simulink model "Mpc_SimMechanics_with_standing"  (R2017b)
settings: Solver=ode45  StartTime=0  StopTime=10  FixedStep=0.0005  EnableMultiTasking=on
InitFcn:
  | isSim = 1;
  | 
  | PreFunctions.CustomInitFcn_with_standing;
  | PreFunctions.simulationInitFcn_with_standing;
undefined symbols (not defined in the file): alpha_x, alpha_y, DiagnosticCodes, DynamicMatrixLibrary, motorPositions, motorVelocities, pelvisPosition, pelvisVelocity, sample_time, X, Y, Z
libraries: sm_lib x170, nesl_utility x75, Contact_Forces_Lib x6, ComponentLibrary x5, xpcrtudplib x2, slrtlib x1
(part 2 of 8)

== system Mpc_SimMechanics_with_standing/Cassie/Cassie Simulation ==
  Bus Element In2 : Inport  PortName=InBus  Element=leftLeg
  Bus Element In3 : Inport  PortName=InBus  Element=rightLeg
  Bus Element In1 : Inport  PortName=InBus  Element=pelvis
  Cassie Left Leg : Subsystem  AncestorBlock=CassieLibrary/Simulation/Cassie Leg  mask{config=Left, motorPositions=motorPositions(1:5), motorVelocities=motorVelocities(1:5)}
      mask prompts: config "Configuration:"; motorPositions "Initial Motor Positions (rad):"; motorVelocities "Initial Motor Velocities (rad/s):"
      mask init:
      | d = CassieDescriptor;
      | bodyIndex = @(s, name) find(arrayfun(@(s) isequal(s.name, name), s));
      | 
      | switch config
      |   case 1 % Left
      |     % Hip Roll
      |     b = d(bodyIndex(d, 'left-hip-roll'));
      |     set_param([gcb, '/Hip Roll Solid'], 'ExtGeomFileName', [b.name '.stl']);
      |     set_param([gcb, '/Hip Roll Solid'], 'Mass', mat2str(b.m));
      |     set_param([gcb, '/Hip Roll Solid'], 'CenterOfMass', mat2str(b.c));
      |     set_param([gcb, '/Hip Roll Solid'], 'MomentsOfInertia', mat2str(b.Ic(1:3)));
      |     set_param([gcb, '/Hip Roll Solid'], 'ProductsOfInertia', mat2str(b.Ic(4:6)));
      |     %set_param([gcb, '/Pelvis to Hip Roll'], 'TranslationCartesianOffset', mat2str(b.r));
      |     %set_param([gcb, '/Pelvis to Hip Roll'], 'RotationMatrix', mat2str(b.R));
      |     
      |     % Hip Yaw
      |     b = d(bodyIndex(d, 'left-hip-yaw'));
      |     set_param([gcb, '/Hip Yaw Solid'], 'ExtGeomFileName', [b.name '.stl']);
      |     set_param([gcb, '/Hip Yaw Solid'], 'Mass', mat2str(b.m));
      |     set_param([gcb, '/Hip Yaw Solid'], 'CenterOfMass', mat2str(b.c));
      |     set_param([gcb, '/Hip Yaw Solid'], 'MomentsOfInertia', mat2str(b.Ic(1:3)));
      |     set_param([gcb, '/Hip Yaw Solid'], 'ProductsOfInertia', mat2str(b.Ic(4:6)));
      |     set_param([gcb, '/Hip Roll to Hip Yaw'], 'TranslationCartesianOffset', mat2str(b.r));
      |     set_param([gcb, '/Hip Roll to Hip Yaw'], 'RotationMatrix', mat2str(b.R));
      |     
      |     % Hip Pitch
      |     b = d(bodyIndex(d, 'left-hip-pitch'));
      |     set_param([gcb, '/Hip Pitch Solid'], 'ExtGeomFileName', [b.name '.stl']);
      |     set_param([gcb, '/Hip Pitch Solid'], 'Mass', mat2str(b.m));
      |     set_param([gcb, '/Hip Pitch Solid'], 'CenterOfMass', mat2str(b.c));
      |     set_param([gcb, '/Hip Pitch Solid'], 'MomentsOfInertia', mat2str(b.Ic(1:3)));
      |     set_param([gcb, '/Hip Pitch Solid'], 'ProductsOfInertia', mat2str(b.Ic(4:6)));
      |     set_param([gcb, '/Hip Yaw to Hip Pitch'], 'TranslationCartesianOffset', mat2str(b.r));
      |     set_param([gcb, '/Hip Yaw to Hip Pitch'], 'RotationMatrix', mat2str(b.R));
      |     
      |     % Achilles Rod
      |     b = d(bodyIndex(d, 'left-achilles-rod'));
      |     set_param([gcb, '/Achilles Rod Solid'], 'ExtGeomFileName', [b.name '.stl']);
      |     set_param([gcb, '/Achilles Rod Solid'], 'Mass', mat2str(b.m));
      |     set_param([gcb, '/Achilles Rod Solid'], 'CenterOfMass', mat2str(b.c));
      |     set_param([gcb, '/Achilles Rod Solid'], 'MomentsOfInertia', mat2str(b.Ic(1:3)));
      |     set_param([gcb, '/Achilles Rod Solid'], 'ProductsOfInertia', mat2str(b.Ic(4:6)));
      |     set_param([gcb, '/Hip Pitch to Achilles Rod'], 'TranslationCartesianOffset', mat2str(b.r));
      |     set_param([gcb, '/Hip Pitch to Achilles Rod'], 'RotationMatrix', mat2str(b.R));
      |     
      |     % Knee
      |     b = d(bodyIndex(d, 'left-knee'));
      |     set_param([gcb, '/Knee Solid'], 'ExtGeomFileName', [b.name '.stl']);
      |     set_param([gcb, '/Knee Solid'], 'Mass', mat2str(b.m));
      |     set_param([gcb, '/Knee Solid'], 'CenterOfMass', mat2str(b.c));
      |     set_param([gcb, '/Knee Solid'], 'MomentsOfInertia', mat2str(b.Ic(1:3)));
      |     set_param([gcb, '/Knee Solid'], 'ProductsOfInertia', mat2str(b.Ic(4:6)));
      |     set_param([gcb, '/Hip Pitch to Knee'], 'TranslationCartesianOffset', mat2str(b.r));
      |     set_param([gcb, '/Hip Pitch to Knee'], 'RotationMatrix', mat2str(b.R));
      |     
      |     % Knee Spring
      |     b = d(bodyIndex(d, 'left-knee-spring'));
      |     set_param([gcb, '/Knee Spring Solid'], 'ExtGeomFileName', [b.name '.stl']);
      |     set_param([gcb, '/Knee Spring Solid'], 'Mass', mat2str(b.m));
      |     set_param([gcb, '/Knee Spring Solid'], 'CenterOfMass', mat2str(b.c));
      |     set_param([gcb, '/Knee Spring Solid'], 'MomentsOfInertia', mat2str(b.Ic(1:3)));
      |     set_param([gcb, '/Knee Spring Solid'], 'ProductsOfInertia', mat2str(b.Ic(4:6)));
      |     set_param([gcb, '/Knee to Knee Spring'], 'TranslationCartesianOffset', mat2str(b.r));
      |     set_param([gcb, '/Knee to Knee Spring'], 'RotationMatrix', mat2str(b.R));
      |     
      |     % Shin
      |     b = d(bodyIndex(d, 'left-shin'));
      |     set_param([gcb, '/Shin Solid'], 'ExtGeomFileName', [b.name '.stl']);
      |     set_param([gcb, '/Shin Solid'], 'Mass', mat2str(b.m));
      |     set_param([gcb, '/Shin Solid'], 'CenterOfMass', mat2str(b.c));
      |     set_param([gcb, '/Shin Solid'], 'MomentsOfInertia', mat2str(b.Ic(1:3)));
      |     set_param([gcb, '/Shin Solid'], 'ProductsOfInertia', mat2str(b.Ic(4:6)));
      |     set_param([gcb, '/Knee to Shin'], 'TranslationCartesianOffset', mat2str(b.r));
      |     set_param([gcb, '/Knee to Shin'], 'RotationMatrix', mat2str(b.R));
      |     
      |     % Tarsus
      |     b = d(bodyIndex(d, 'left-tarsus'));
      |     set_param([gcb, '/Tarsus Solid'], 'ExtGeomFileName', [b.name '.stl']);
      |     set_param([gcb, '/Tarsus Solid'], 'Mass', mat2str(b.m));
      |     set_param([gcb, '/Tarsus Solid'], 'CenterOfMass', mat2str(b.c));
      |     set_param([gcb, '/Tarsus Solid'], 'MomentsOfInertia', mat2str(b.Ic(1:3)));
      |     set_param([gcb, '/Tarsus Solid'], 'ProductsOfInertia', mat2str(b.Ic(4:6)));
      |     set_param([gcb, '/Shin to Tarsus'], 'TranslationCartesianOffset', mat2str(b.r));
      |     set_param([gcb, '/Shin to Tarsus'], 'RotationMatrix', mat2str(b.R));
      |     
      |     % Heel Spring
      |     b = d(bodyIndex(d, 'left-heel-spring'));
      |     set_param([gcb, '/Heel Spring Solid'], 'ExtGeomFileName', [b.name '.stl']);
      |     set_param([gcb, '/Heel Spring Solid'], 'Mass', mat2str(b.m));
      |     set_param([gcb, '/Heel Spring Solid'], 'CenterOfMass', mat2str(b.c));
      |     set_param([gcb, '/Heel Spring Solid'], 'MomentsOfInertia', mat2str(b.Ic(1:3)));
      |     set_param([gcb, '/Heel Spring Solid'], 'ProductsOfInertia', mat2str(b.Ic(4:6)));
      |     set_param([gcb, '/Tarsus to Heel Spring'], 'TranslationCartesianOffset', mat2str(b.r));
      |     set_param([gcb, '/Tarsus to Heel Spring'], 'RotationMatrix', mat2str(b.R));
      |     
      |     % Foot Crank
      |     b = d(bodyIndex(d, 'left-foot-crank'));
      |     set_param([gcb, '/Foot Crank Solid'], 'ExtGeomFileName', [b.name '.stl']);
      |     set_param([gcb, '/Foot Crank Solid'], 'Mass', mat2str(b.m));
      |     set_param([gcb, '/Foot Crank Solid'], 'CenterOfMass', mat2str(b.c));
      |     set_param([gcb, '/Foot Crank Solid'], 'MomentsOfInertia', mat2str(b.Ic(1:3)));
      |     set_param([gcb, '/Foot Crank Solid'], 'ProductsOfInertia', mat2str(b.Ic(4:6)));
      |     set_param([gcb, '/Tarsus to Foot Crank'], 'TranslationCartesianOffset', mat2str(b.r));
      |     set_param([gcb, '/Tarsus to Foot Crank'], 'RotationMatrix', mat2str(b.R));
      |     
      |     % Plantar Rod
      |     b = d(bodyIndex(d, 'left-plantar-rod'));
      |     set_param([gcb, '/Plantar Rod Solid'], 'ExtGeomFileName', [b.name '.stl']);
      |     set_param([gcb, '/Plantar Rod Solid'], 'Mass', mat2str(b.m));
      |     set_param([gcb, '/Plantar Rod Solid'], 'CenterOfMass', mat2str(b.c));
      |     set_param([gcb, '/Plantar Rod Solid'], 'MomentsOfInertia', mat2str(b.Ic(1:3)));
      |     set_param([gcb, '/Plantar Rod Solid'], 'ProductsOfInertia', mat2str(b.Ic(4:6)));
      |     set_param([gcb, '/Foot Crank to Plantar Rod'], 'TranslationCartesianOffset', mat2str(b.r));
      |     set_param([gcb, '/Foot Crank to Plantar Rod'], 'RotationMatrix', mat2str(b.R));
      |     
      |     % Foot
      |     b = d(bodyIndex(d, 'left-foot'));
      |     set_param([gcb, '/Foot Solid'], 'ExtGeomFileName', [b.name '.stl']);
      |     set_param([gcb, '/Foot Solid'], 'Mass', mat2str(b.m));
      |     set_param([gcb, '/Foot Solid'], 'CenterOfMass', mat2str(b.c));
      |     set_param([gcb, '/Foot Solid'], 'MomentsOfInertia', mat2str(b.Ic(1:3)));
      |     set_param([gcb, '/Foot Solid'], 'ProductsOfInertia', mat2str(b.Ic(4:6)));
      |     set_param([gcb, '/Tarsus to Foot'], 'TranslationCartesianOffset', mat2str(b.r));
      |     set_param([gcb, '/Tarsus to Foot'], 'RotationMatrix', mat2str(b.R));
      |     
      |     % Foot Pin
      |     %b = d(bodyIndex(d, 'left-foot-pin'));
      |     set_param([gcb, '/Foot to Foot Pin'], 'TranslationCartesianOffset', mat2str([0.055 0 0.00776]));
      |     set_param([gcb, '/Foot to Foot Pin'], 'RotationMatrix', mat2str(eye(3)));
      |     
      |     % Midfoot
      |     %b = d(bodyIndex(d, 'left-mid-foot'));
      |     set_param([gcb, '/Foot to Midfoot'], 'TranslationCartesianOffset', mat2str([0.01762 0.05219 0]));
      |     set_param([gcb, '/Foot to Midfoot'], 'RotationMatrix', mat2str([-0.766044443118978 0 -0.642787609686539;0.642787609686539 0 -0.766044443118978;0 -1 0]));
      |     
      |   case 2 % Right
      |     % Hip Roll
      |     b = d(bodyIndex(d, 'right-hip-roll'));
      |     set_param([gcb, '/Hip Roll Solid'], 'ExtGeomFileName', [b.name '.stl']);
      |     set_param([gcb, '/Hip Roll Solid'], 'Mass', mat2str(b.m));
      |     set_param([gcb, '/Hip Roll Solid'], 'CenterOfMass', mat2str(b.c));
      |     set_param([gcb, '/Hip Roll Solid'], 'MomentsOfInertia', mat2str(b.Ic(1:3)));
      |     set_param([gcb, '/Hip Roll Solid'], 'ProductsOfInertia', mat2str(b.Ic(4:6)));
      |     %set_param([gcb, '/Pelvis to Hip Roll'], 'TranslationCartesianOffset', mat2str(b.r));
      |     %set_param([gcb, '/Pelvis to Hip Roll'], 'RotationMatrix', mat2str(b.R));
      |     
      |     % Hip Yaw
      |     b = d(bodyIndex(d, 'right-hip-yaw'));
      |     set_param([gcb, '/Hip Yaw Solid'], 'ExtGeomFileName', [b.name '.stl']);
      |     set_param([gcb, '/Hip Yaw Solid'], 'Mass', mat2str(b.m));
      |     set_param([gcb, '/Hip Yaw Solid'], 'CenterOfMass', mat2str(b.c));
      |     set_param([gcb, '/Hip Yaw Solid'], 'MomentsOfInertia', mat2str(b.Ic(1:3)));
      |     set_param([gcb, '/Hip Yaw Solid'], 'ProductsOfInertia', mat2str(b.Ic(4:6)));
      |     set_param([gcb, '/Hip Roll to Hip Yaw'], 'TranslationCartesianOffset', mat2str(b.r));
      |     set_param([gcb, '/Hip Roll to Hip Yaw'], 'RotationMatrix', mat2str(b.R));
      |     
      |     % Hip Pitch
      |     b = d(bodyIndex(d, 'right-hip-pitch'));
      |     set_param([gcb, '/Hip Pitch Solid'], 'ExtGeomFileName', [b.name '.stl']);
      |     set_param([gcb, '/Hip Pitch Solid'], 'Mass', mat2str(b.m));
      |     set_param([gcb, '/Hip Pitch Solid'], 'CenterOfMass', mat2str(b.c));
      |     set_param([gcb, '/Hip Pitch Solid'], 'MomentsOfInertia', mat2str(b.Ic(1:3)));
      |     set_param([gcb, '/Hip Pitch Solid'], 'ProductsOfInertia', mat2str(b.Ic(4:6)));
      |     set_param([gcb, '/Hip Yaw to Hip Pitch'], 'TranslationCartesianOffset', mat2str(b.r));
      |     set_param([gcb, '/Hip Yaw to Hip Pitch'], 'RotationMatrix', mat2str(b.R));
      |     
      |     % Achilles Rod
      |     b = d(bodyIndex(d, 'right-achilles-rod'));
      |     set_param([gcb, '/Achilles Rod Solid'], 'ExtGeomFileName', [b.name '.stl']);
      |     set_param([gcb, '/Achilles Rod Solid'], 'Mass', mat2str(b.m));
      |     set_param([gcb, '/Achilles Rod Solid'], 'CenterOfMass', mat2str(b.c));
      |     set_param([gcb, '/Achilles Rod Solid'], 'MomentsOfInertia', mat2str(b.Ic(1:3)));
      |     set_param([gcb, '/Achilles Rod Solid'], 'ProductsOfInertia', mat2str(b.Ic(4:6)));
      |     set_param([gcb, '/Hip Pitch to Achilles Rod'], 'TranslationCartesianOffset', mat2str(b.r));
      |     set_param([gcb, '/Hip Pitch to Achilles Rod'], 'RotationMatrix', mat2str(b.R));
      |     
      |     % Knee
      |     b = d(bodyIndex(d, 'right-knee'));
      |     set_param([gcb, '/Knee Solid'], 'ExtGeomFileName', [b.name '.stl']);
      |     set_param([gcb, '/Knee Solid'], 'Mass', mat2str(b.m));
      |     set_param([gcb, '/Knee Solid'], 'CenterOfMass', mat2str(b.c));
      |     set_param([gcb, '/Knee Solid'], 'MomentsOfInertia', mat2str(b.Ic(1:3)));
      |     set_param([gcb, '/Knee Solid'], 'ProductsOfInertia', mat2str(b.Ic(4:6)));
      |     set_param([gcb, '/Hip Pitch to Knee'], 'TranslationCartesianOffset', mat2str(b.r));
      |     set_param([gcb, '/Hip Pitch to Knee'], 'RotationMatrix', mat2str(b.R));
      |     
      |     % Knee Spring
      |     b = d(bodyIndex(d, 'right-knee-spring'));
      |     set_param([gcb, '/Knee Spring Solid'], 'ExtGeomFileName', [b.name '.stl']);
      |     set_param([gcb, '/Knee Spring Solid'], 'Mass', mat2str(b.m));
      |     set_param([gcb, '/Knee Spring Solid'], 'CenterOfMass', mat2str(b.c));
      |     set_param([gcb, '/Knee Spring Solid'], 'MomentsOfInertia', mat2str(b.Ic(1:3)));
      |     set_param([gcb, '/Knee Spring Solid'], 'ProductsOfInertia', mat2str(b.Ic(4:6)));
      |     set_param([gcb, '/Knee to Knee Spring'], 'TranslationCartesianOffset', mat2str(b.r));
      |     set_param([gcb, '/Knee to Knee Spring'], 'RotationMatrix', mat2str(b.R));
      |     
      |     % Shin
      |     b = d(bodyIndex(d, 'right-shin'));
      |     set_param([gcb, '/Shin Solid'], 'ExtGeomFileName', [b.name '.stl']);
      |     set_param([gcb, '/Shin Solid'], 'Mass', mat2str(b.m));
      |     set_param([gcb, '/Shin Solid'], 'CenterOfMass', mat2str(b.c));
      |     set_param([gcb, '/Shin Solid'], 'MomentsOfInertia', mat2str(b.Ic(1:3)));
      |     set_param([gcb, '/Shin Solid'], 'ProductsOfInertia', mat2str(b.Ic(4:6)));
      |     set_param([gcb, '/Knee to Shin'], 'TranslationCartesianOffset', mat2str(b.r));
      |     set_param([gcb, '/Knee to Shin'], 'RotationMatrix', mat2str(b.R));
      |     
      |     % Tarsus
      |     b = d(bodyIndex(d, 'right-tarsus'));
      |     set_param([gcb, '/Tarsus Solid'], 'ExtGeomFileName', [b.name '.stl']);
      |     set_param([gcb, '/Tarsus Solid'], 'Mass', mat2str(b.m));
      |     set_param([gcb, '/Tarsus Solid'], 'CenterOfMass', mat2str(b.c));
      |     set_param([gcb, '/Tarsus Solid'], 'MomentsOfInertia', mat2str(b.Ic(1:3)));
      |     set_param([gcb, '/Tarsus Solid'], 'ProductsOfInertia', mat2str(b.Ic(4:6)));
      |     set_param([gcb, '/Shin to Tarsus'], 'TranslationCartesianOffset', mat2str(b.r));
      |     set_param([gcb, '/Shin to Tarsus'], 'RotationMatrix', mat2str(b.R));
      |     
      |     % Heel Spring
      |     b = d(bodyIndex(d, 'right-heel-spring'));
      |     set_param([gcb, '/Heel Spring Solid'], 'ExtGeomFileName', [b.name '.stl']);
      |     set_param([gcb, '/Heel Spring Solid'], 'Mass', mat2str(b.m));
      |     set_param([gcb, '/Heel Spring Solid'], 'CenterOfMass', mat2str(b.c));
      |     set_param([gcb, '/Heel Spring Solid'], 'MomentsOfInertia', mat2str(b.Ic(1:3)));
      |     set_param([gcb, '/Heel Spring Solid'], 'ProductsOfInertia', mat2str(b.Ic(4:6)));
      |     set_param([gcb, '/Tarsus to Heel Spring'], 'TranslationCartesianOffset', mat2str(b.r));
      |     set_param([gcb, '/Tarsus to Heel Spring'], 'RotationMatrix', mat2str(b.R));
      |     
      |     % Foot Crank
      |     b = d(bodyIndex(d, 'right-foot-crank'));
      |     set_param([gcb, '/Foot Crank Solid'], 'ExtGeomFileName', [b.name '.stl']);
      |     set_param([gcb, '/Foot Crank Solid'], 'Mass', mat2str(b.m));
      |     set_param([gcb, '/Foot Crank Solid'], 'CenterOfMass', mat2str(b.c));
      |     set_param([gcb, '/Foot Crank Solid'], 'MomentsOfInertia', mat2str(b.Ic(1:3)));
      |     set_param([gcb, '/Foot Crank Solid'], 'ProductsOfInertia', mat2str(b.Ic(4:6)));
      |     set_param([gcb, '/Tarsus to Foot Crank'], 'TranslationCartesianOffset', mat2str(b.r));
      |     set_param([gcb, '/Tarsus to Foot Crank'], 'RotationMatrix', mat2str(b.R));
      |     
      |     % Plantar Rod
      |     b = d(bodyIndex(d, 'right-plantar-rod'));
      |     set_param([gcb, '/Plantar Rod Solid'], 'ExtGeomFileName', [b.name '.stl']);
      |     set_param([gcb, '/Plantar Rod Solid'], 'Mass', mat2str(b.m));
      |     set_param([gcb, '/Plantar Rod Solid'], 'CenterOfMass', mat2str(b.c));
      |     set_param([gcb, '/Plantar Rod Solid'], 'MomentsOfInertia', mat2str(b.Ic(1:3)));
      |     set_param([gcb, '/Plantar Rod Solid'], 'ProductsOfInertia', mat2str(b.Ic(4:6)));
      |     set_param([gcb, '/Foot Crank to Plantar Rod'], 'TranslationCartesianOffset', mat2str(b.r));
      |     set_param([gcb, '/Foot Crank to Plantar Rod'], 'RotationMatrix', mat2str(b.R));
      |     
      |     % Foot
      |     b = d(bodyIndex(d, 'right-foot'));
      |     set_param([gcb, '/Foot Solid'], 'ExtGeomFileName', [b.name '.stl']);
      |     set_param([gcb, '/Foot Solid'], 'Mass', mat2str(b.m));
      |     set_param([gcb, '/Foot Solid'], 'CenterOfMass', mat2str(b.c));
      |     set_param([gcb, '/Foot Solid'], 'MomentsOfInertia', mat2str(b.Ic(1:3)));
      |     set_param([gcb, '/Foot Solid'], 'ProductsOfInertia', mat2str(b.Ic(4:6)));
      |     set_param([gcb, '/Tarsus to Foot'], 'TranslationCartesianOffset', mat2str(b.r));
      |     set_param([gcb, '/Tarsus to Foot'], 'RotationMatrix', mat2str(b.R));
      |     
      |     % Foot Pin
      |     %b = d(bodyIndex(d, 'right-foot-pin'));
      |     set_param([gcb, '/Foot to Foot Pin'], 'TranslationCartesianOffset', mat2str([0.055 0 -0.00776]));
      |     set_param([gcb, '/Foot to Foot Pin'], 'RotationMatrix', mat2str(eye(3)));
      |     
      |     % Midfoot
      |     %b = d(bodyIndex(d, 'right-mid-foot'));
      |     set_param([gcb, '/Foot to Midfoot'], 'TranslationCartesianOffset', mat2str([0.01762 0.05219 0]));
      |     set_param([gcb, '/Foot to Midfoot'], 'RotationMatrix', mat2str([-0.766044443118978 0 -0.642787609686539;0.642787609686539 0 -0.766044443118978;0 -1 0]));
      | end % switch
      | 
      | % Check if block is not in library model
      | if ~bdIsLibrary(bdroot)
      |   % Construct discrete filter for velocity estimation
      |   dt = str2num(get_param(bdroot, 'FixedStep'));
      |   filter1 = ButterworthFilter(2);
      |   filter1.setTimeConstant(0.003, dt);
      |   filter2 = BackwardDifferencingFilter(2);
      |   filter2.setSampleTime(dt);
      |   filter3 = Filter(filter1, filter2, 'cascade');
      |   [a, b] = filter3.getCoefficients;
      |   
      |   % Set discrete filter coefficients    
      |   set_param([gcb '/Shin Filter'], 'a', mat2str(a));
      |   set_param([gcb '/Shin Filter'], 'b', mat2str(b));
      |   set_param([gcb '/Tarsus Filter'], 'a', mat2str(a));
      |   set_param([gcb '/Tarsus Filter'], 'b', mat2str(b));
      |   set_param([gcb '/Foot Filter'], 'a', mat2str(a));
      |   set_param([gcb '/Foot Filter'], 'b', mat2str(b));
      | end % if
      mask TypeOptions config: Left | Right
  Cassie Pelvis : Subsystem  AncestorBlock=CassieLibrary/Simulation/Cassie Pelvis
  Cassie Right Leg : Subsystem  AncestorBlock=CassieLibrary/Simulation/Cassie Leg  mask{config=Right, motorPositions=motorPositions(6:10), motorVelocities=motorVelocities(6:10)}
      mask prompts: config "Configuration:"; motorPositions "Initial Motor Positions (rad):"; motorVelocities "Initial Motor Velocities (rad/s):"
      mask init: same as Mpc_SimMechanics_with_standing/Cassie/Cassie Simulation/Cassie Left Leg
      mask TypeOptions config: Left | Right
  Constant : Constant  Value=true
  Constant1 : Constant  Value=DiagnosticCodes(zeros(4,1))
  Manual Switch : ManualSwitch
  Manual Switch1 : ManualSwitch
  Mux : Mux  Inputs=9
  World : Subsystem  AncestorBlock=ComponentLibrary/Simulation/World
  Bus Element Out4 : Outport  PortName=OutBus  Element=pelvis
  Bus Element Out2 : Outport  PortName=OutBus  Element=leftLeg
  Bus Element Out3 : Outport  PortName=OutBus  Element=rightLeg
  Bus Element Out1 : Outport  PortName=OutBus  Element=isCalibrated
  Bus Element Out5 : Outport  PortName=OutBus  Element=messages
  perfect measurement : Outport  Port=2
  wires:
  Constant1/1 -> Bus Element Out5/1
  Constant/1 -> Bus Element Out1/1
  Bus Element In1/1 -> Cassie Pelvis/1(InBus)
  Cassie Right Leg/1(OutBus) -> Bus Element Out3/1
  Bus Element In2/1 -> Cassie Left Leg/1(InBus)
  Cassie Left Leg/1(OutBus) -> Bus Element Out2/1
  Bus Element In3/1 -> Cassie Right Leg/1(InBus)
  Cassie Pelvis/1(OutBus) -> Bus Element Out4/1
  Cassie Pelvis/2(LinearAccelerator) -> Mux/1
  Cassie Pelvis/3(Quaternion) -> Mux/2
  Cassie Pelvis/4(AngularVelocity) -> Mux/3
  Cassie Left Leg/2(pos) -> Mux/5
  Cassie Right Leg/2(pos) -> Mux/6
  Cassie Left Leg/3(vel) -> Mux/8
  Cassie Right Leg/3(vel) -> Mux/9
  Mux/1 -> perfect measurement/1
  World/1(base_pos) -> Manual Switch/2
  World/2(base_vel) -> Manual Switch1/2
  Cassie Pelvis/6(IMU_vel) -> Manual Switch1/1
  Cassie Pelvis/5(IMU_pos) -> Manual Switch/1
  Manual Switch/1 -> Mux/4
  Manual Switch1/1 -> Mux/7
  connections:
  World/RConn1 -- Cassie Pelvis/LConn1
  Cassie Left Leg/LConn1 -- Cassie Pelvis/RConn1
  Cassie Pelvis/RConn2 -- Cassie Right Leg/LConn1

== system Mpc_SimMechanics_with_standing/Controller/file_scopes ==
  In1 : Inport
  Data Bus Selector : BusSelector  OutputSignals=t,s,q,dq,u,x0_next_goal,x0_next_tgd_goal,dxf_next_goal,dxf_next_tgd_goal,dxf_this_stTD0,y0_next_goal,y0_next_tgd_goal,dyf_this_tgd,dyf_this_stTD0,dyf_next_tgd_goal,px_com,py_com,pz_com,vx_com,vy_com,vz_com,ufp_sol_rel_st_x,ufp_sol_rel_st_y,ufp_sol_rel_com_x,ufp_sol_rel_com_y,Vx_tgd_des,Vy_tgd_des,Lx_tgd_des,Ly_tgd_des,rp_stToe,rv_stToe,Lx_stToe_kf,Ly_stToe_kf,stanceLeg,stTD0,tg_direction,kx_body,kx_world,ky_body,ky_world,mu,T_period
  Scope 1 : slrtlib/Displays and Logging/Scope   scopeno=5  scopetype=File  autostart=on  viewmode=Graphical redraw  formatstr='%15.6f'  grid=on  ylimits=[0,0]  nosamples=250  noprepostsamples=0  interleave=1  triggermode=FreeRun  triggersignal=1  trigsignalfromport=off  triggerlevel=0.0  triggerslope=Either  triggerscope=1  triggersample=0  filename=DATA.dat  mode=Commit  writesize=512*8  autorestart=on  dynamicfilemode=off  maxwritefilesize=1024^3
  Vector Concatenate : Concatenate  NumInputs=42
  wires:
  Data Bus Selector/6 -> Vector Concatenate/6  "<x0_next_goal>"
  Data Bus Selector/41 -> Vector Concatenate/41  "<mu>"
  Data Bus Selector/26 -> Vector Concatenate/26  "<Vx_tgd_des>"
  Vector Concatenate/1 -> Scope 1/1
  Data Bus Selector/5 -> Vector Concatenate/5  "<u>"
  Data Bus Selector/42 -> Vector Concatenate/42  "<T_period>"
  Data Bus Selector/27 -> Vector Concatenate/27  "<Vy_tgd_des>"
  Data Bus Selector/12 -> Vector Concatenate/12  "<y0_next_tgd_goal>"
  Data Bus Selector/31 -> Vector Concatenate/31  "<rv_stToe>"
  Data Bus Selector/33 -> Vector Concatenate/33  "<Ly_stToe_kf>"
  Data Bus Selector/9 -> Vector Concatenate/9  "<dxf_next_tgd_goal>"
  Data Bus Selector/4 -> Vector Concatenate/4  "<dq>"
  Data Bus Selector/38 -> Vector Concatenate/38  "<kx_world>"
  Data Bus Selector/40 -> Vector Concatenate/40  "<ky_world>"
  Data Bus Selector/36 -> Vector Concatenate/36  "<tg_direction>"
  Data Bus Selector/17 -> Vector Concatenate/17  "<py_com>"
  Data Bus Selector/16 -> Vector Concatenate/16  "<px_com>"
  Data Bus Selector/25 -> Vector Concatenate/25  "<ufp_sol_rel_com_y>"
  Data Bus Selector/39 -> Vector Concatenate/39  "<ky_body>"
  Data Bus Selector/35 -> Vector Concatenate/35  "<stTD0>"
  Data Bus Selector/28 -> Vector Concatenate/28  "<Lx_tgd_des>"
  Data Bus Selector/24 -> Vector Concatenate/24  "<ufp_sol_rel_com_x>"
  Data Bus Selector/2 -> Vector Concatenate/2  "<s>"
  Data Bus Selector/37 -> Vector Concatenate/37  "<kx_body>"
  Data Bus Selector/23 -> Vector Concatenate/23  "<ufp_sol_rel_st_y>"
  In1/1 -> Data Bus Selector/1
  Data Bus Selector/20 -> Vector Concatenate/20  "<vy_com>"
  Data Bus Selector/29 -> Vector Concatenate/29  "<Ly_tgd_des>"
  Data Bus Selector/22 -> Vector Concatenate/22  "<ufp_sol_rel_st_x>"
  Data Bus Selector/32 -> Vector Concatenate/32  "<Lx_stToe_kf>"
  Data Bus Selector/21 -> Vector Concatenate/21  "<vz_com>"
  Data Bus Selector/8 -> Vector Concatenate/8  "<dxf_next_goal>"
  Data Bus Selector/10 -> Vector Concatenate/10  "<dxf_this_stTD0>"
  Data Bus Selector/7 -> Vector Concatenate/7  "<x0_next_tgd_goal>"
  Data Bus Selector/30 -> Vector Concatenate/30  "<rp_stToe>"
  Data Bus Selector/19 -> Vector Concatenate/19  "<vx_com>"
  Data Bus Selector/13 -> Vector Concatenate/13  "<dyf_this_tgd>"
  Data Bus Selector/34 -> Vector Concatenate/34  "<stanceLeg>"
  Data Bus Selector/14 -> Vector Concatenate/14  "<dyf_this_stTD0>"
  Data Bus Selector/15 -> Vector Concatenate/15  "<dyf_next_tgd_goal>"
  Data Bus Selector/3 -> Vector Concatenate/3  "<q>"
  Data Bus Selector/1 -> Vector Concatenate/1  "<t>"
  Data Bus Selector/18 -> Vector Concatenate/18  "<pz_com>"
  Data Bus Selector/11 -> Vector Concatenate/11  "<y0_next_goal>"

== system Mpc_SimMechanics_with_standing/Controller/mpc_lip_footplacement ==
  SlrtToLinux : Inport  OutDataTypeStr=Bus: SlrtToLinuxDataBus
  Constant : Constant  Value=64+2
  MATLAB System : MATLABSystem  System=SlrtToLinuxDataBusToBytes  SimulateUsing=Code generation
      mask Type: SlrtToLinuxDataBusToBytes
      mask Display: disp('SlrtToLinuxDataBusToBytes');
  MATLAB System1 : MATLABSystem  System=BytesToLinuxToSlrtDataBus  SimulateUsing=Code generation
      mask Type: BytesToLinuxToSlrtDataBus
      mask Display: disp('BytesToLinuxToSlrtDataBus');
  MATLAB System3 : MATLABSystem  System=ProcessUdpPacket  heartbeatInterval=0.01  dataLength=20  SimulateUsing=Code generation
      mask Type: ProcessUdpPacket
      mask Display:
      | disp('ProcessUdpPacket');
      | port_label('input',1,'UDP Data');
      | port_label('input',2,'Length');
      | port_label('output',1,'Log');
      | port_label('output',2,'Header');
      | port_label('output',3,'Data');
  Rate Transition : RateTransition  InitialCondition=zeros(20,1)  OutPortSampleTime=sample_time
  Rate Transition1 : RateTransition  InitialCondition=zeros(64,1)  OutPortSampleTime=udp_sample_time
  To Workspace : ToWorkspace  VariableName=simout  SaveFormat=Timeseries  SampleTime=-1
  UDP Receive : xpcrtudplib/UDP Receive  ipAddressVal=Use host-target connection  localPort=udp_local_port  rcvWidth=20+2  rcvFmAny=off  fmAddress=udp_linux_ip_address  maxUDPQueue=8  sampleTime=udp_sample_time
      settings: SourceProductName=Simulink Real-Time
  UDP Send : xpcrtudplib/UDP Send  ipAddressVal=Use host-target connection  localPort=udp_local_port  toAddress=udp_linux_ip_address  toPort=udp_remote_port  sampleTime=udp_sample_time
      settings: SourceProductName=Simulink Real-Time  SourceProductBaseCode=XP
  Vector Concatenate : Concatenate
  "LinuxToSlrt " : Outport
  wires:
  UDP Receive/1 -> MATLAB System3/1
  Constant/1 -> UDP Send/2
  MATLAB System1/1 -> "LinuxToSlrt "/1
  Vector Concatenate/1 -> UDP Send/1
  MATLAB System3/2 -> Vector Concatenate/1
  MATLAB System3/1 -> To Workspace/1
  UDP Receive/2 -> MATLAB System3/2
  MATLAB System/1 -> Rate Transition1/1
  Rate Transition1/1 -> Vector Concatenate/2
  Rate Transition/1 -> MATLAB System1/1
  MATLAB System3/3 -> Rate Transition/1
  SlrtToLinux/1 -> MATLAB System/1

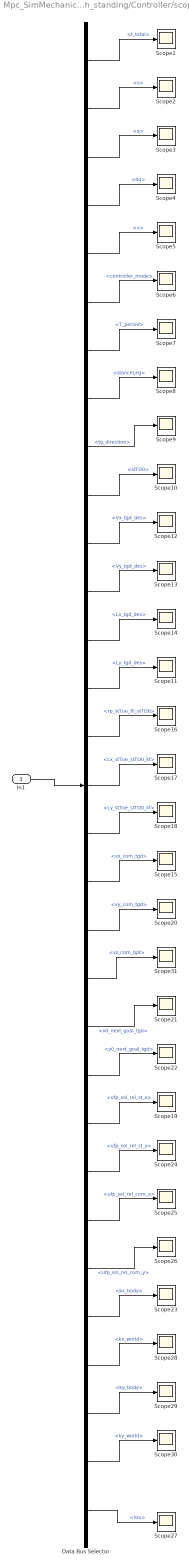
== system Mpc_SimMechanics_with_standing/Controller/scopes ==
  In1 : Inport
  Data Bus Selector : BusSelector  OutputSignals=t_total,s,q,dq,u,controller_mode,T_period,stanceLeg,tg_direction,stTD0,Vx_tgd_des,Vy_tgd_des,Lx_tgd_des,Ly_tgd_des,rp_stToe_fil_stTD0,Lx_stToe_stTD0_kf,Ly_stToe_stTD0_kf,vx_com_tgd,vy_com_tgd,vz_com_tgd,x0_next_goal_tgd,y0_next_goal_tgd,ufp_sol_rel_st_x,ufp_sol_rel_st_y,ufp_sol_rel_com_x,ufp_sol_rel_com_y,kx_body,kx_world,ky_body,ky_world,mu
  Scope{1..31} (31 alike) : Scope
  wires:
  In1/1 -> Data Bus Selector/1
  Data Bus Selector/1 -> Scope1/1  "<t_total>"
  Data Bus Selector/2 -> Scope2/1  "<s>"
  Data Bus Selector/3 -> Scope3/1  "<q>"
  Data Bus Selector/4 -> Scope4/1  "<dq>"
  Data Bus Selector/5 -> Scope5/1  "<u>"
  Data Bus Selector/6 -> Scope6/1  "<controller_mode>"
  Data Bus Selector/7 -> Scope7/1  "<T_period>"
  Data Bus Selector/8 -> Scope8/1  "<stanceLeg>"
  Data Bus Selector/10 -> Scope10/1  "<stTD0>"
  Data Bus Selector/9 -> Scope9/1  "<tg_direction>"
  Data Bus Selector/11 -> Scope12/1  "<Vx_tgd_des>"
  Data Bus Selector/12 -> Scope13/1  "<Vy_tgd_des>"
  Data Bus Selector/13 -> Scope14/1  "<Lx_tgd_des>"
  Data Bus Selector/14 -> Scope11/1  "<Ly_tgd_des>"
  Data Bus Selector/15 -> Scope16/1  "<rp_stToe_fil_stTD0>"
  Data Bus Selector/16 -> Scope17/1  "<Lx_stToe_stTD0_kf>"
  Data Bus Selector/17 -> Scope18/1  "<Ly_stToe_stTD0_kf>"
  Data Bus Selector/18 -> Scope15/1  "<vx_com_tgd>"
  Data Bus Selector/19 -> Scope20/1  "<vy_com_tgd>"
  Data Bus Selector/21 -> Scope21/1  "<x0_next_goal_tgd>"
  Data Bus Selector/22 -> Scope22/1  "<y0_next_goal_tgd>"
  Data Bus Selector/23 -> Scope19/1  "<ufp_sol_rel_st_x>"
  Data Bus Selector/24 -> Scope24/1  "<ufp_sol_rel_st_y>"
  Data Bus Selector/25 -> Scope25/1  "<ufp_sol_rel_com_x>"
  Data Bus Selector/26 -> Scope26/1  "<ufp_sol_rel_com_y>"
  Data Bus Selector/27 -> Scope23/1  "<kx_body>"
  Data Bus Selector/28 -> Scope28/1  "<kx_world>"
  Data Bus Selector/29 -> Scope29/1  "<ky_body>"
  Data Bus Selector/30 -> Scope30/1  "<ky_world>"
  Data Bus Selector/31 -> Scope27/1  "<mu>"
  Data Bus Selector/20 -> Scope31/1  "<vz_com_tgd>"
